simulink model "p4simulink"  (R2025a)
settings: Solver=ode45  StartTime=0.0  StopTime=10.0  MaxStep=0.01  RelTol=1e-3
values from neighbouring files (symbols this model uses):
  k = 100    [practica4.m]
  m = 10    [practica4.m]
settings Model: LastModifiedBy=ismae

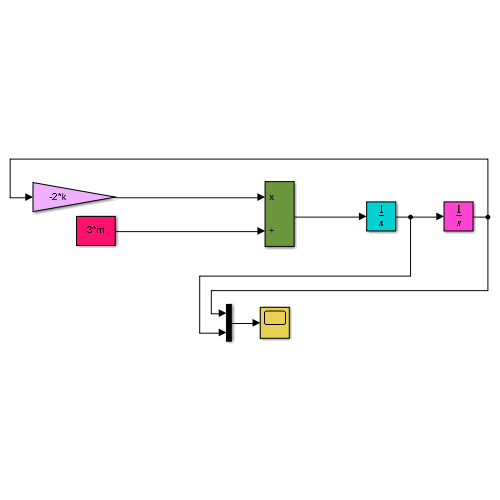
[thumbnail: Simulink's stored preview of the top-level diagram]
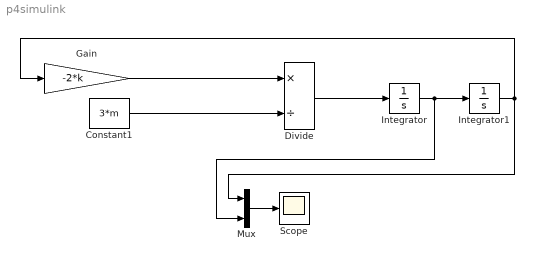
== system p4simulink ==
  Constant1 : Constant  Value=3*m
  Divide : Product  Inputs=*/
  Gain : Gain  Gain=-2*k
  Integrator : Integrator  InitialCondition=2
  Integrator1 : Integrator
  Mux : Mux  Inputs=2
  Scope : Scope
      settings: ActiveDisplayYMinimum=-1.6336531783701909  ActiveDisplayYMaximum=2.685102895487923
  wires:
  Integrator/1 -> Mux/2, Integrator1/1
  Constant1/1 -> Divide/2
  Divide/1 -> Integrator/1
  Gain/1 -> Divide/1
  Mux/1 -> Scope/1
  Integrator1/1 -> Gain/1, Mux/1
